simulink model "NoLinealSolo"  (R2020b)
settings: Solver=VariableStepAuto  StartTime=0.0  StopTime=10  RelTol=1e-3
values from neighbouring files (symbols this model uses):
  a0 = 0.001505    [params.m]
  a2 = -0.000055    (= -5.5e-05)    [params.m]
  alfa_o = 0    [params.m]
  g = 9.81    [params.m]
  I = m1*r1^2+m2*r2^2+m3*r3^2    (= 0.0018475)    [params.m]
  m1 = 0.031    [params.m]
  m2 = 0.019    [params.m]
  m3 = 0.02    [params.m]
  p1 = 0.052    [params.m]
  p2 = -0.0036    [params.m]
  r1 = 0.19    [params.m]
  r2 = 0.16    [params.m]
  r3 = 0.11    [params.m]
  vo = 3.855    [params.m]
settings Model: Creator=bou  LastModifiedBy=bou
settings SolverCC: AlgebraicLoopSolver=LineSearch

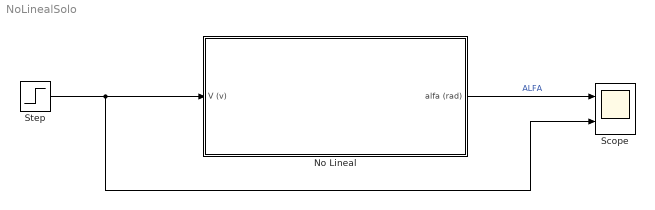
== system NoLinealSolo ==
  No Lineal : Subsystem
  Scope : Scope  NumInputPorts=2
  Step : Step  Time=0  Before=vo  After=vo  SampleTime=0
  wires:
  Step/1 -> Scope/2, No Lineal/1(V (v))
  No Lineal/1(alfa (rad)) -> Scope/1  "ALFA"

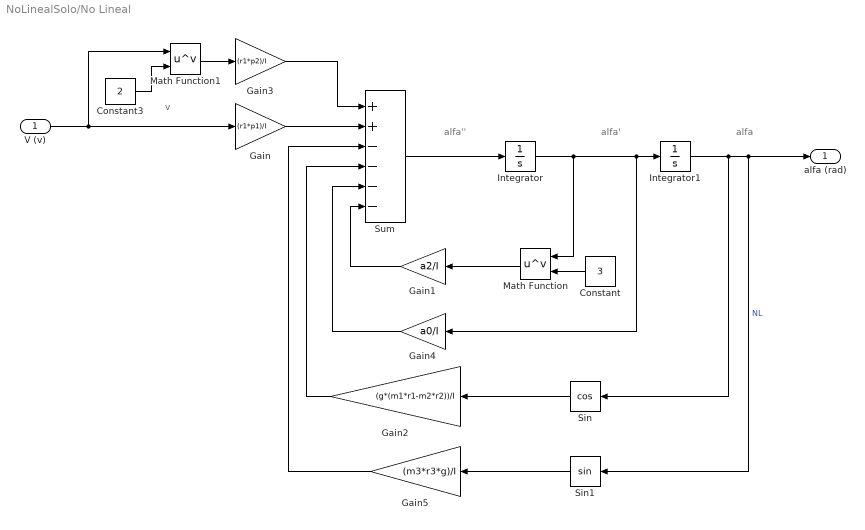
== system NoLinealSolo/No Lineal ==
  note: v
  note: alfa
  note: alfa'
  note: alfa''
  V (v) : Inport
  Constant : Constant  Value=3
  Constant3 : Constant  Value=2
  Gain : Gain  Gain=(r1*p1)/I
  Gain1 : Gain  Gain=a2/I
  Gain2 : Gain  Gain=(g*(m1*r1-m2*r2))/I
  Gain3 : Gain  Gain=(r1*p2)/I
  Gain4 : Gain  Gain=a0/I
  Gain5 : Gain  Gain=(m3*r3*g)/I
  Integrator : Integrator  InitialCondition=alfa_o
  Integrator1 : Integrator  InitialCondition=alfa_o
  Math Function : Math  Operator=pow  SaturateOnIntegerOverflow=on
  Math Function1 : Math  Operator=pow  SaturateOnIntegerOverflow=on
  Sin : Trigonometry  Operator=cos
  Sin1 : Trigonometry
  Sum : Sum  Inputs=++----
  alfa (rad) : Outport
  wires:
  Sin/1 -> Gain2/1
  Gain5/1 -> Sum/3
  Constant3/1 -> Math Function1/2
  Integrator1/1 -> alfa (rad)/1, Sin1/1, Sin/1  "NL"
  Gain3/1 -> Sum/1
  Gain2/1 -> Sum/4
  V (v)/1 -> Math Function1/1, Gain/1
  Gain/1 -> Sum/2
  Sum/1 -> Integrator/1
  Sin1/1 -> Gain5/1
  Math Function1/1 -> Gain3/1
  Gain4/1 -> Sum/5
  Constant/1 -> Math Function/2
  Integrator/1 -> Integrator1/1, Gain4/1, Math Function/1
  Math Function/1 -> Gain1/1
  Gain1/1 -> Sum/6
